simulink model "untitled1"  (R2017a)
settings: Solver=VariableStepAuto  StartTime=0.0  StopTime=10.0  RelTol=1e-3
libraries: mpclib x1, simulink x1
settings Model: Creator=gunge  LastModifiedBy=gunge

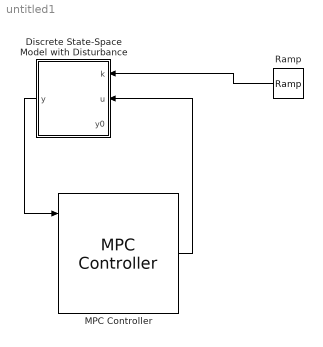
== system untitled1 ==
  Discrete State-Space Model with Disturbance : MATLAB Function  TreatAsAtomicUnit=on
  MPC Controller : mpclib/MPC Controller  SCDEnableBlockLinearizationSpecification=on  is_multiple=0  enable_value=0  return_u0=off  ref_from_ws=off  ref_signal_name=[]  ref_preview=off  md_from_ws=off  md_signal_name=[]  md_preview=off  from_project=off  project_file=MPCtask.mat  md_inport=on  mv_inport=off  cost_outport=off  return_sequence=off  return_qpstatus=off  return_state=off  state_inport=off  lims_inport=off  ywt_inport=off  is_designfromscratch=0  uwt_inport=off  duwt_inport=off  rhoeps_inport=off  uref_inport=off  n_ts=1  n_mv=1  n_md=1  n_ud=0  n_mo=1  n_uo=0  BlockDataType=double  SampleTimeInherited=off  switch_inport=off
  Ramp : simulink/Sources/Ramp  slope=1  start=0  X0=1
  wires:
  Discrete State-Space Model with Disturbance/1(y) -> MPC Controller/1
  MPC Controller/1 -> Discrete State-Space Model with Disturbance/2(u)
  Ramp/1 -> Discrete State-Space Model with Disturbance/1(k)

== matlab function untitled1/Discrete State-Space Model with Disturbance ==
  data: k input; u input; y output; y0 input
function y = fcn(k,u,y0)

A = [   0.461, -0.0503,   0,   0;
       0.0745,   0.548,   0,   0;
      0.00474,  0.0752, 1.0,   0;
         2.23,    1.01, 3.1, 1.0];
    
B = [   0.134;
        4.34;
        0.238;
        3.7];
    
C = [ 0 0 0 1 ];

D = [0];

Ts = 0.1;

% Initial Condition
x0 = [ 0;0;0;y0 ];

t(:,1) = x0

t(:,k+1) = A * t(:,k) + B * u;
y = C * t(:,k) + D * u;
